simulink model "S4_LP_SCR_bypass_2018b"  (R2018b)
settings: Solver=VariableStepAuto  StartTime=0.0  StopTime=20000  RelTol=1e-3
undefined symbols (not defined in the file or in its folder): sigbuilder_block
libraries: fl_lib x70, sh_lib x49, nesl_utility x29
(part 1 of 2)
settings Model: Creator=USER  LastModifiedBy=USER
settings DataIOCC: ReturnWorkspaceOutputs=on
settings DebuggingCC: UnconnectedInputMsg=none  UnconnectedOutputMsg=none  UnconnectedLineMsg=none  SFMachineParentedDataDiag=error
settings SimscapeCC: SimscapeLogType=all

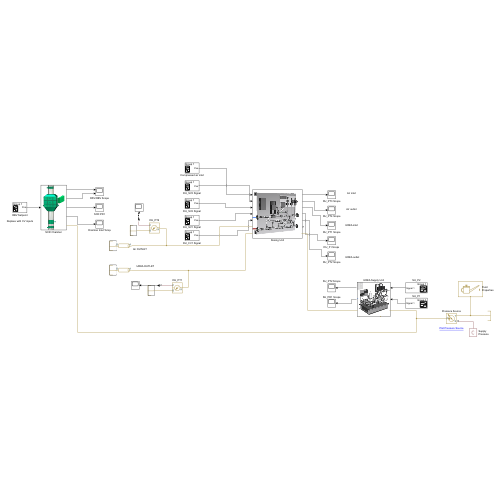
[thumbnail: Simulink's stored preview of the top-level diagram]
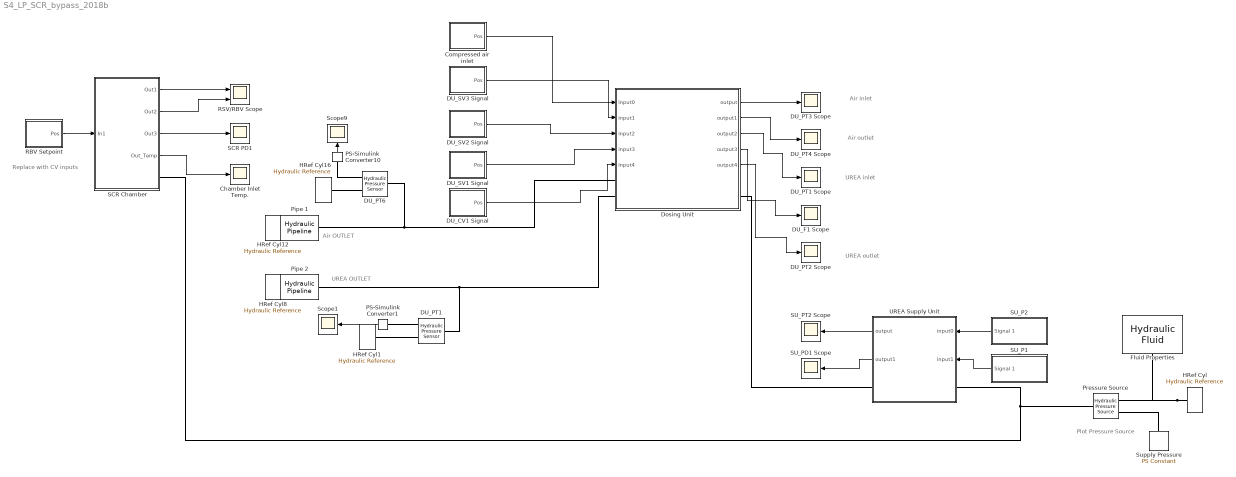
== system S4_LP_SCR_bypass_2018b ==
  note: Air inlet
  note: UREA inlet
  note: UREA outlet
  note: Air outlet
  note: Air OUTLET
  note: Plot Pressure Source
  note: UREA OUTLET
  note: Replace with CV inputs
  Chamber Inlet Temp. : Scope
  Compressed air inlet : Subsystem  Tag=STV Subsys  LoadFcn=sigbuilder_block('load');  StartFcn=sigbuilder_block('start');  StopFcn=sigbuilder_block('stop');  ClipboardFcn=sigbuilder_block('clipboard');  mask(Sigbuilder block){tuvar=[0:10]}
      mask help: Sigbuilder GUI
      mask init:
      | if ~strcmp(get_param(bdroot(gcbh),'SimulationStatus'),'stopped') tuvar = sigbuilder_block('maskInit'); end
      settings: CopyFcn=sigbuilder_block('copy');  DeleteFcn=sigbuilder_block('delete');  ModelCloseFcn=sigbuilder_block('modelClose');  PreSaveFcn=sigbuilder_block('preSave');  PauseFcn=sigbuilder_block('pause')  ContinueFcn=sigbuilder_block('continue')  NameChangeFcn=sigbuilder_block('namechange');  OpenFcn=sigbuilder_block('open',[0 0 787.5 524.25 ]);  CloseFcn=sigbuilder_block('close');
      mask Display: plot(0, 0, 100, 100,[2, 2, 32, 32, 2], [68, 8, 8, 68, 68],[32, 2], [38, 38], [32, 19, 2],[53, 60, 44], [32, 17, 17, 2],[16, 16, 31, 31]);txt = getActiveGroup(gcbh);text(2, 100, txt,'verticalAlignment', 'top');
  DU_CV1 Signal : Subsystem  Tag=STV Subsys  LoadFcn=sigbuilder_block('load');  StartFcn=sigbuilder_block('start');  StopFcn=sigbuilder_block('stop');  ClipboardFcn=sigbuilder_block('clipboard');  mask(Sigbuilder block){tuvar=[0:10]}
      mask help: Sigbuilder GUI
      mask init:
      | if ~strcmp(get_param(bdroot(gcbh),'SimulationStatus'),'stopped') tuvar = sigbuilder_block('maskInit'); end
      settings: CopyFcn=sigbuilder_block('copy');  DeleteFcn=sigbuilder_block('delete');  ModelCloseFcn=sigbuilder_block('modelClose');  PreSaveFcn=sigbuilder_block('preSave');  PauseFcn=sigbuilder_block('pause')  ContinueFcn=sigbuilder_block('continue')  NameChangeFcn=sigbuilder_block('namechange');  OpenFcn=sigbuilder_block('open',[0 0 787.5 524.25 ]);  CloseFcn=sigbuilder_block('close');
      mask Display: plot(0, 0, 100, 100,[2, 2, 32, 32, 2], [68, 8, 8, 68, 68],[32, 2], [38, 38], [32, 19, 2],[53, 60, 44], [32, 17, 17, 2],[16, 16, 31, 31]);txt = getActiveGroup(gcbh);text(2, 100, txt,'verticalAlignment', 'top');
  DU_F1 Scope : Scope
  DU_PT1 : fl_lib/Hydraulic/Hydraulic Sensors/Hydraulic Pressure Sensor
      settings: SourceProductBaseCode=PW,SS,VE
  DU_PT1 Scope : Scope
  DU_PT2 Scope : Scope
  DU_PT3 Scope : Scope
  DU_PT4 Scope : Scope
  DU_PT6 : fl_lib/Hydraulic/Hydraulic Sensors/Hydraulic Pressure Sensor
      settings: SourceProductBaseCode=PW,SS,VE
  DU_SV1 Signal : Subsystem  Tag=STV Subsys  LoadFcn=sigbuilder_block('load');  StartFcn=sigbuilder_block('start');  StopFcn=sigbuilder_block('stop');  ClipboardFcn=sigbuilder_block('clipboard');  mask(Sigbuilder block){tuvar=[0:10]}
      mask help: Sigbuilder GUI
      mask init:
      | if ~strcmp(get_param(bdroot(gcbh),'SimulationStatus'),'stopped') tuvar = sigbuilder_block('maskInit'); end
      settings: CopyFcn=sigbuilder_block('copy');  DeleteFcn=sigbuilder_block('delete');  ModelCloseFcn=sigbuilder_block('modelClose');  PreSaveFcn=sigbuilder_block('preSave');  PauseFcn=sigbuilder_block('pause')  ContinueFcn=sigbuilder_block('continue')  NameChangeFcn=sigbuilder_block('namechange');  OpenFcn=sigbuilder_block('open',[0 0 787.5 524.25 ]);  CloseFcn=sigbuilder_block('close');
      mask Display: plot(0, 0, 100, 100,[2, 2, 32, 32, 2], [68, 8, 8, 68, 68],[32, 2], [38, 38], [32, 19, 2],[53, 60, 44], [32, 17, 17, 2],[16, 16, 31, 31]);txt = getActiveGroup(gcbh);text(2, 100, txt,'verticalAlignment', 'top');
  DU_SV2 Signal : Subsystem  Tag=STV Subsys  LoadFcn=sigbuilder_block('load');  StartFcn=sigbuilder_block('start');  StopFcn=sigbuilder_block('stop');  ClipboardFcn=sigbuilder_block('clipboard');  mask(Sigbuilder block){tuvar=[0:10]}
      mask help: Sigbuilder GUI
      mask init:
      | if ~strcmp(get_param(bdroot(gcbh),'SimulationStatus'),'stopped') tuvar = sigbuilder_block('maskInit'); end
      settings: CopyFcn=sigbuilder_block('copy');  DeleteFcn=sigbuilder_block('delete');  ModelCloseFcn=sigbuilder_block('modelClose');  PreSaveFcn=sigbuilder_block('preSave');  PauseFcn=sigbuilder_block('pause')  ContinueFcn=sigbuilder_block('continue')  NameChangeFcn=sigbuilder_block('namechange');  OpenFcn=sigbuilder_block('open',[0 0 787.5 524.25 ]);  CloseFcn=sigbuilder_block('close');
      mask Display: plot(0, 0, 100, 100,[2, 2, 32, 32, 2], [68, 8, 8, 68, 68],[32, 2], [38, 38], [32, 19, 2],[53, 60, 44], [32, 17, 17, 2],[16, 16, 31, 31]);txt = getActiveGroup(gcbh);text(2, 100, txt,'verticalAlignment', 'top');
  DU_SV3 Signal : Subsystem  Tag=STV Subsys  LoadFcn=sigbuilder_block('load');  StartFcn=sigbuilder_block('start');  StopFcn=sigbuilder_block('stop');  ClipboardFcn=sigbuilder_block('clipboard');  mask(Sigbuilder block){tuvar=[0:10]}
      mask help: Sigbuilder GUI
      mask init:
      | if ~strcmp(get_param(bdroot(gcbh),'SimulationStatus'),'stopped') tuvar = sigbuilder_block('maskInit'); end
      settings: CopyFcn=sigbuilder_block('copy');  DeleteFcn=sigbuilder_block('delete');  ModelCloseFcn=sigbuilder_block('modelClose');  PreSaveFcn=sigbuilder_block('preSave');  PauseFcn=sigbuilder_block('pause')  ContinueFcn=sigbuilder_block('continue')  NameChangeFcn=sigbuilder_block('namechange');  OpenFcn=sigbuilder_block('open',[1483.5 44.25 813 562.5 ]);  CloseFcn=sigbuilder_block('close');
      mask Display: plot(0, 0, 100, 100,[2, 2, 32, 32, 2], [68, 8, 8, 68, 68],[32, 2], [38, 38], [32, 19, 2],[53, 60, 44], [32, 17, 17, 2],[16, 16, 31, 31]);txt = getActiveGroup(gcbh);text(2, 100, txt,'verticalAlignment', 'top');
  Dosing Unit : Subsystem
      mask Display: image('DosingUnit.png')
  Fluid Properties : sh_lib/Hydraulic Utilities/Hydraulic Fluid  Tag=Factory Generic  SelFluid=2  SysTemp=40  TrapAir=0.001  ViscDerFactor=1  range_error=2
  HRef Cyl{,1,8,12,16} (5 alike) : fl_lib/Hydraulic/Hydraulic Elements/Hydraulic Reference  Tag=Factory Generic
      settings: SourceProductBaseCode=PW,SS,VE
  PS-Simulink Converter1 : nesl_utility/PS-Simulink Converter  PhysicalDomain=network_engine_domain  SubClassName=ps_output  LeftPortType=input  RightPortType=output  PseudoPeriodic=off  Frequencies=[]  VectorFormat=inherit  Unit=inherit  AffineConversion=off
      settings: SourceProductBaseCode=SS,PW,VE
  PS-Simulink Converter10 : nesl_utility/PS-Simulink Converter  PhysicalDomain=network_engine_domain  SubClassName=ps_output  LeftPortType=input  RightPortType=output  PseudoPeriodic=off  Frequencies=[]  VectorFormat=inherit  Unit=inherit  AffineConversion=off
      settings: SourceProductBaseCode=SS,PW,VE
  Pipe 1 : sh_lib/Pipelines/Hydraulic Pipeline  Tag=Factory Generic  cs_type=1  d_in=0.1 m  area=1e-04 m^2  D_h=0.0112 m  s_factor=64  length=5 m  length_ad=1 m  roughness=1.5e-05 m  Re_lam=2e+03  Re_turb=4e+03  wall_type=1  pr_r_coef=2e-10 m/Pa  time_const=0.008 s  k_sh=1.4  initial_pressure=0 Pa
      settings: SourceProductBaseCode=SH  InternalSimscapePortConfiguration="{\"Bottom\":[],\"Left\":[{\"id\":\"A\",\"label\":\"A\",\"type\":\"foundation.hydraulic.hydraulic\"}],\"Right\":[{\"id\":\"B\",\"label\":\"B\",\"type\":\"foundation.hydraulic.hydraulic\"}],\"Top\":[]}"
  Pipe 2 : sh_lib/Pipelines/Hydraulic Pipeline  Tag=Factory Generic  cs_type=1  d_in=0.1 m  area=1e-04 m^2  D_h=0.0112 m  s_factor=64  length=1 m  length_ad=1 m  roughness=1.5e-05 m  Re_lam=2e+03  Re_turb=4e+03  wall_type=1  pr_r_coef=2e-10 m/Pa  time_const=0.008 s  k_sh=1.4  initial_pressure=0 Pa
      settings: SourceProductBaseCode=SH  InternalSimscapePortConfiguration="{\"Bottom\":[],\"Left\":[{\"id\":\"A\",\"label\":\"A\",\"type\":\"foundation.hydraulic.hydraulic\"}],\"Right\":[{\"id\":\"B\",\"label\":\"B\",\"type\":\"foundation.hydraulic.hydraulic\"}],\"Top\":[]}"
  Pressure Source : fl_lib/Hydraulic/Hydraulic Sources/Hydraulic Pressure Source  Tag=Factory Generic
      settings: SourceProductBaseCode=PW,SS,VE  InternalSimscapePortConfiguration="{\"Bottom\":[],\"Left\":[{\"id\":\"P\",\"label\":\"P\",\"type\":\"foundation.hydraulic.hydraulic\"}],\"Right\":[{\"id\":\"S\",\"label\":\"S\",\"type\":\"input\"},{\"id\":\"T\",\"label\":\"T\",\"type\":\"foundation.hydraulic.hydraulic\"}],\"Top\":[]}"
  RBV Setpoint : Subsystem  Tag=STV Subsys  LoadFcn=sigbuilder_block('load');  StartFcn=sigbuilder_block('start');  StopFcn=sigbuilder_block('stop');  ClipboardFcn=sigbuilder_block('clipboard');  mask(Sigbuilder block){tuvar=[0:10]}
      mask help: Sigbuilder GUI
      mask init:
      | if ~strcmp(get_param(bdroot(gcbh),'SimulationStatus'),'stopped') tuvar = sigbuilder_block('maskInit'); end
      settings: CopyFcn=sigbuilder_block('copy');  DeleteFcn=sigbuilder_block('delete');  ModelCloseFcn=sigbuilder_block('modelClose');  PreSaveFcn=sigbuilder_block('preSave');  PauseFcn=sigbuilder_block('pause')  ContinueFcn=sigbuilder_block('continue')  NameChangeFcn=sigbuilder_block('namechange');  OpenFcn=sigbuilder_block('open',[0 0 787.5 524.25 ]);  CloseFcn=sigbuilder_block('close');
      mask Display: plot(0, 0, 100, 100,[2, 2, 32, 32, 2], [68, 8, 8, 68, 68],[32, 2], [38, 38], [32, 19, 2],[53, 60, 44], [32, 17, 17, 2],[16, 16, 31, 31]);txt = getActiveGroup(gcbh);text(2, 100, txt,'verticalAlignment', 'top');
  RSV/RBV Scope : Scope  NumInputPorts=2
  SCR Chamber : Subsystem
      mask Display: image('SCRChamber.png')
  SCR PD1 : Scope
  SU_P1 : Subsystem  Tag=STV Subsys  LoadFcn=sigbuilder_block('load');  StartFcn=sigbuilder_block('start');  StopFcn=sigbuilder_block('stop');  ClipboardFcn=sigbuilder_block('clipboard');  mask(Sigbuilder block){tuvar=[0:10]}
      mask help: Simulink:masks:SigbuilderBlock_MD
      mask init:
      | if ~strcmp(get_param(bdroot(gcbh),'SimulationStatus'),'stopped') tuvar = sigbuilder_block('maskInit'); end
      settings: CopyFcn=sigbuilder_block('copy');  DeleteFcn=sigbuilder_block('delete');  ModelCloseFcn=sigbuilder_block('modelClose');  PreSaveFcn=sigbuilder_block('preSave');  PauseFcn=sigbuilder_block('pause');  ContinueFcn=sigbuilder_block('continue');  NameChangeFcn=sigbuilder_block('namechange');  OpenFcn=sigbuilder_block('open',[0 0 787.5 524.25 ]);  CloseFcn=sigbuilder_block('close');
      mask Display: plot(0, 0, 100, 100,[2, 2, 32, 32, 2], [68, 8, 8, 68, 68],[32, 2], [38, 38], [32, 19, 2],[53, 60, 44], [32, 17, 17, 2],[16, 16, 31, 31]);txt = getActiveGroup(gcbh);text(2, 100, txt,'verticalAlignment', 'top');
  SU_P2 : Subsystem  Tag=STV Subsys  LoadFcn=sigbuilder_block('load');  StartFcn=sigbuilder_block('start');  StopFcn=sigbuilder_block('stop');  ClipboardFcn=sigbuilder_block('clipboard');  mask(Sigbuilder block){tuvar=[0:10]}
      mask help: Simulink:masks:SigbuilderBlock_MD
      mask init:
      | if ~strcmp(get_param(bdroot(gcbh),'SimulationStatus'),'stopped') tuvar = sigbuilder_block('maskInit'); end
      settings: CopyFcn=sigbuilder_block('copy');  DeleteFcn=sigbuilder_block('delete');  ModelCloseFcn=sigbuilder_block('modelClose');  PreSaveFcn=sigbuilder_block('preSave');  PauseFcn=sigbuilder_block('pause');  ContinueFcn=sigbuilder_block('continue');  NameChangeFcn=sigbuilder_block('namechange');  OpenFcn=sigbuilder_block('open',[0 0 787.5 524.25 ]);  CloseFcn=sigbuilder_block('close');
      mask Display: plot(0, 0, 100, 100,[2, 2, 32, 32, 2], [68, 8, 8, 68, 68],[32, 2], [38, 38], [32, 19, 2],[53, 60, 44], [32, 17, 17, 2],[16, 16, 31, 31]);txt = getActiveGroup(gcbh);text(2, 100, txt,'verticalAlignment', 'top');
  SU_PD1 Scope : Scope
  SU_PT2 Scope : Scope
  Scope1 : Scope
  Scope9 : Scope
  Supply Pressure : fl_lib/Physical Signals/Sources/PS Constant  constant=7 Pa
      settings: SourceProductBaseCode=PW,SS,VE
  UREA Supply Unit : Subsystem
      mask Display: image('UreaSupplyUnit.png')
  wires:
  SU_P2/1(Signal 1) -> UREA Supply Unit/1(input0)
  SU_P1/1(Signal 1) -> UREA Supply Unit/2(input1)
  UREA Supply Unit/1(output) -> SU_PT2 Scope/1
  UREA Supply Unit/2(output1) -> SU_PD1 Scope/1
  Compressed air inlet/1(Pos) -> Dosing Unit/1(input0)
  DU_SV3 Signal/1(Pos) -> Dosing Unit/2(input1)
  DU_SV2 Signal/1(Pos) -> Dosing Unit/3(input2)
  DU_SV1 Signal/1(Pos) -> Dosing Unit/4(input3)
  DU_CV1 Signal/1(Pos) -> Dosing Unit/5(input4)
  Dosing Unit/1(output) -> DU_PT3 Scope/1
  Dosing Unit/2(output1) -> DU_PT4 Scope/1
  Dosing Unit/3(output2) -> DU_PT1 Scope/1
  Dosing Unit/4(output3) -> DU_F1 Scope/1
  Dosing Unit/5(output4) -> DU_PT2 Scope/1
  PS-Simulink Converter10/1 -> Scope9/1
  PS-Simulink Converter1/1 -> Scope1/1
  RBV Setpoint/1(Pos) -> SCR Chamber/1(In1)
  SCR Chamber/1(Out1) -> RSV/RBV Scope/1
  SCR Chamber/2(Out2) -> RSV/RBV Scope/2
  SCR Chamber/3(Out3) -> SCR PD1/1
  SCR Chamber/4(Out_Temp) -> Chamber Inlet Temp./1
  connections:
  HRef Cyl/LConn1 -- Fluid Properties/RConn1 -- Pressure Source/RConn2
  Supply Pressure/RConn1 -- Pressure Source/RConn1
  Pipe 1/RConn1 -- HRef Cyl12/LConn1
  Pipe 2/RConn1 -- HRef Cyl8/LConn1
  Pipe 1/LConn1 -- DU_PT6/LConn1 -- Dosing Unit/LConn1
  Dosing Unit/LConn2 -- Pipe 2/LConn1 -- DU_PT1/LConn1
  UREA Supply Unit/RConn1 -- Dosing Unit/RConn2
  PS-Simulink Converter10/LConn1 -- DU_PT6/RConn2
  HRef Cyl16/LConn1 -- DU_PT6/RConn1
  HRef Cyl1/LConn1 -- DU_PT1/RConn1
  PS-Simulink Converter1/LConn1 -- DU_PT1/RConn2
  Pressure Source/LConn1 -- SCR Chamber/RConn1 -- UREA Supply Unit/LConn1

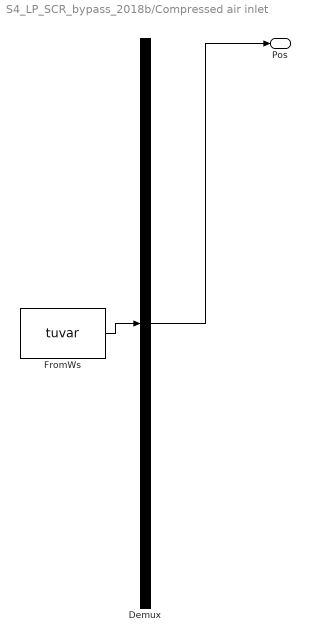
== system S4_LP_SCR_bypass_2018b/Compressed air inlet ==
  Demux : Demux  Tag=STV Demux  Outputs=1
      settings: DisplayOption=none
  FromWs : FromWorkspace  Tag=STV FromWs  VariableName=tuvar
      SigBuilderData=|
      | common.afterFinalStr = 'Extrapolate'
      | common.sampleTime = 0
      | dataSet.timeRange = [0 20000]
      | dataSet.name = 'Group 1'
      | sbobj.Groups.Name = 'Group 1'
      | sbobj.Groups.Signals.Name = 'Pos'
      | sbobj.Groups.Signals.XData = [0 20000]
      | sbobj.Groups.Signals.YData = [1 1]
      | sbobj.Groups.TimeRange = [0 20000]
  Pos : Outport  Tag=STV Outport  VectorParamsAs1DForOutWhenUnconnected=off
  wires:
  Demux/1 -> Pos/1
  FromWs/1 -> Demux/1

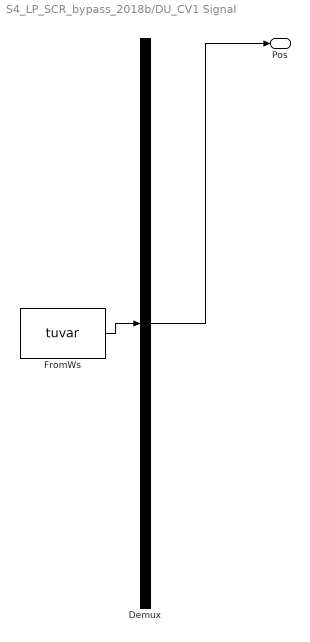
== system S4_LP_SCR_bypass_2018b/DU_CV1 Signal ==
  Demux : Demux  Tag=STV Demux  Outputs=1
      settings: DisplayOption=none
  FromWs : FromWorkspace  Tag=STV FromWs  VariableName=tuvar
      SigBuilderData=|
      | common.afterFinalStr = 'Extrapolate'
      | common.sampleTime = 0
      | dataSet.timeRange = [0 20000]
      | dataSet.name = 'Group 1'
      | sbobj.Groups.Name = 'Group 1'
      | sbobj.Groups.Signals.Name = 'Pos'
      | sbobj.Groups.Signals.XData = [0 8720 8720 9040 9040 11820 11820 12436 12436 20000]
      | sbobj.Groups.Signals.YData = [0 0 1 1 -0.005 0 1 1 0 0]
      | sbobj.Groups.TimeRange = [0 20000]
  Pos : Outport  Tag=STV Outport  VectorParamsAs1DForOutWhenUnconnected=off
  wires:
  Demux/1 -> Pos/1
  FromWs/1 -> Demux/1

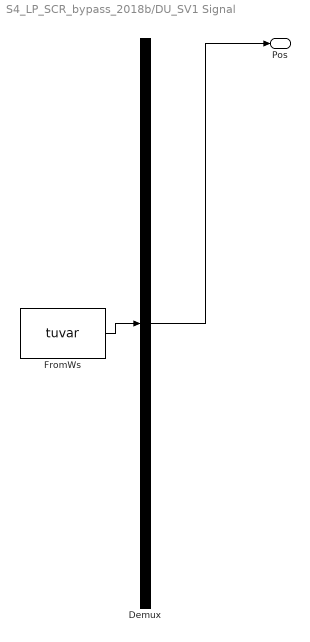
== system S4_LP_SCR_bypass_2018b/DU_SV1 Signal ==
  Demux : Demux  Tag=STV Demux  Outputs=1
      settings: DisplayOption=none
  FromWs : FromWorkspace  Tag=STV FromWs  VariableName=tuvar
      SigBuilderData=|
      | common.afterFinalStr = 'Extrapolate'
      | common.sampleTime = 0
      | dataSet.timeRange = [0 20000]
      | dataSet.name = 'Group 1'
      | sbobj.Groups.Name = 'Group 1'
      | sbobj.Groups.Signals.Name = 'Pos'
      | sbobj.Groups.Signals.XData = [0 9040 9040 11820 11820 20000]
      | sbobj.Groups.Signals.YData = [0 0 1 1 0 0]
      | sbobj.Groups.TimeRange = [0 20000]
  Pos : Outport  Tag=STV Outport  VectorParamsAs1DForOutWhenUnconnected=off
  wires:
  Demux/1 -> Pos/1
  FromWs/1 -> Demux/1

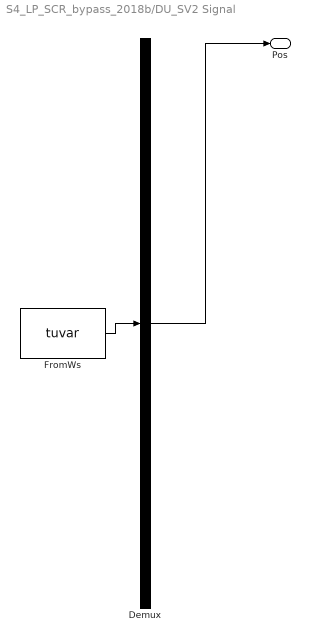
== system S4_LP_SCR_bypass_2018b/DU_SV2 Signal ==
  Demux : Demux  Tag=STV Demux  Outputs=1
      settings: DisplayOption=none
  FromWs : FromWorkspace  Tag=STV FromWs  VariableName=tuvar
      SigBuilderData=|
      | common.afterFinalStr = 'Extrapolate'
      | common.sampleTime = 0
      | dataSet.timeRange = [0 20000]
      | dataSet.name = 'Group 1'
      | sbobj.Groups.Name = 'Group 1'
      | sbobj.Groups.Signals.Name = 'Pos'
      | sbobj.Groups.Signals.XData = [0 8720 8720 9040 9040 11820 11820 12436 12436 20000]
      | sbobj.Groups.Signals.YData = [0 0 1 1 -0.005 0 1 1 0 0]
      | sbobj.Groups.TimeRange = [0 20000]
  Pos : Outport  Tag=STV Outport  VectorParamsAs1DForOutWhenUnconnected=off
  wires:
  Demux/1 -> Pos/1
  FromWs/1 -> Demux/1

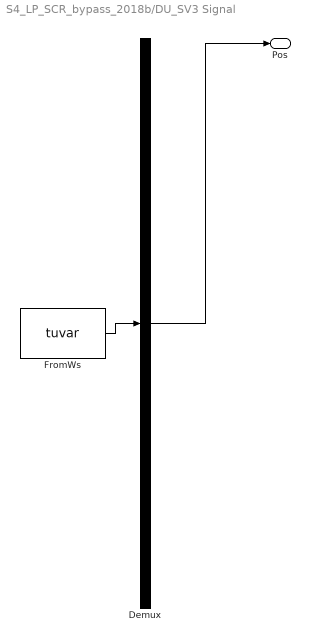
== system S4_LP_SCR_bypass_2018b/DU_SV3 Signal ==
  Demux : Demux  Tag=STV Demux  Outputs=1
      settings: DisplayOption=none
  FromWs : FromWorkspace  Tag=STV FromWs  VariableName=tuvar
      SigBuilderData=|
      | common.afterFinalStr = 'Extrapolate'
      | common.sampleTime = 0
      | dataSet.timeRange = [0 20000]
      | dataSet.name = 'Group 1'
      | sbobj.Groups.Name = 'Group 1'
      | sbobj.Groups.Signals.Name = 'Pos'
      | sbobj.Groups.Signals.XData = [0 8696 8696 12251 12251 20000]
      | sbobj.Groups.Signals.YData = [0 0 1 1 0 0]
      | sbobj.Groups.TimeRange = [0 20000]
  Pos : Outport  Tag=STV Outport  VectorParamsAs1DForOutWhenUnconnected=off
  wires:
  Demux/1 -> Pos/1
  FromWs/1 -> Demux/1

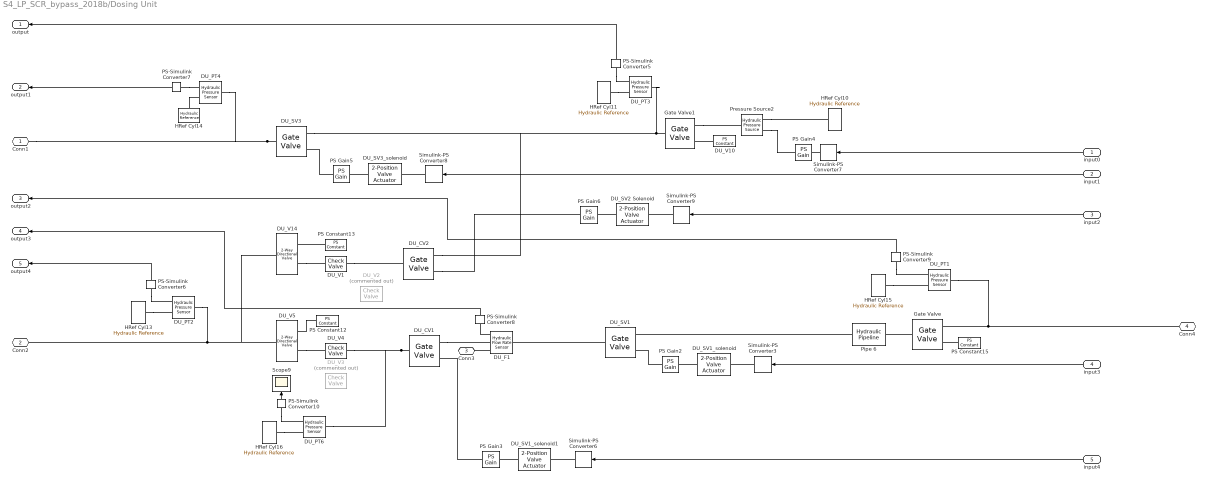
== system S4_LP_SCR_bypass_2018b/Dosing Unit ==
  input0 : Inport
  input1 : Inport  Port=2
  input2 : Inport  Port=3
  input3 : Inport  Port=4
  input4 : Inport  Port=5
  DU_CV1 : sh_lib/Valves/Flow Control Valves/Gate Valve  d_gate=0.1 m  x_0=0 m  C_d=1e3  A_leak=500 m^2  lam_spec=1  B_lam=0.999  Re_cr=10
      settings: SourceProductBaseCode=SH  InternalSimscapePortConfiguration="{\"Bottom\":[],\"Left\":[{\"id\":\"S\",\"label\":\"S\",\"type\":\"input\"},{\"id\":\"A\",\"label\":\"A\",\"type\":\"foundation.hydraulic.hydraulic\"}],\"Right\":[{\"id\":\"B\",\"label\":\"B\",\"type\":\"foundation.hydraulic.hydraulic\"}],\"Top\":[]}"
  DU_CV2 : sh_lib/Valves/Flow Control Valves/Gate Valve  d_gate=0.1 m  x_0=0 m  C_d=1e3  A_leak=500 m^2  lam_spec=1  B_lam=0.999  Re_cr=10
      settings: SourceProductBaseCode=SH  InternalSimscapePortConfiguration="{\"Bottom\":[],\"Left\":[{\"id\":\"S\",\"label\":\"S\",\"type\":\"input\"},{\"id\":\"A\",\"label\":\"A\",\"type\":\"foundation.hydraulic.hydraulic\"}],\"Right\":[{\"id\":\"B\",\"label\":\"B\",\"type\":\"foundation.hydraulic.hydraulic\"}],\"Top\":[]}"
  DU_F1 : fl_lib/Hydraulic/Hydraulic Sensors/Hydraulic Flow Rate Sensor
      settings: SourceProductBaseCode=PW,SS,VE
  DU_PT{1..4,6} (5 alike) : fl_lib/Hydraulic/Hydraulic Sensors/Hydraulic Pressure Sensor
      settings: SourceProductBaseCode=PW,SS,VE
  DU_SV1 : sh_lib/Valves/Flow Control Valves/Gate Valve  d_gate=0.1 m  x_0=0 m  C_d=500  A_leak=1e-20 m^2  lam_spec=1  B_lam=0.999  Re_cr=10
      settings: SourceProductBaseCode=SH  InternalSimscapePortConfiguration="{\"Bottom\":[],\"Left\":[{\"id\":\"S\",\"label\":\"S\",\"type\":\"input\"},{\"id\":\"A\",\"label\":\"A\",\"type\":\"foundation.hydraulic.hydraulic\"}],\"Right\":[{\"id\":\"B\",\"label\":\"B\",\"type\":\"foundation.hydraulic.hydraulic\"}],\"Top\":[]}"
  DU_SV1_solenoid : sh_lib/Valves/Valve Actuators/2-Position Valve Actuator  stroke=1 m  t_on=2 s  t_off=2 s  act_signal=1e-20  init_position=0  act_orientation=1
      settings: SourceProductBaseCode=SH  InternalSimscapePortConfiguration="{\"Bottom\":[],\"Left\":[{\"id\":\"C\",\"label\":\"\",\"type\":\"input\"}],\"Right\":[{\"id\":\"P\",\"label\":\"\",\"type\":\"output\"}],\"Top\":[]}"
  DU_SV1_solenoid1 : sh_lib/Valves/Valve Actuators/2-Position Valve Actuator  stroke=1 m  t_on=2 s  t_off=2 s  act_signal=1e-20  init_position=0  act_orientation=1
      settings: SourceProductBaseCode=SH  InternalSimscapePortConfiguration="{\"Bottom\":[],\"Left\":[{\"id\":\"C\",\"label\":\"\",\"type\":\"input\"}],\"Right\":[{\"id\":\"P\",\"label\":\"\",\"type\":\"output\"}],\"Top\":[]}"
  DU_SV2 Solenoid : sh_lib/Valves/Valve Actuators/2-Position Valve Actuator  stroke=1 m  t_on=2 s  t_off=2 s  act_signal=1e-20  init_position=0  act_orientation=1
      settings: SourceProductBaseCode=SH  InternalSimscapePortConfiguration="{\"Bottom\":[],\"Left\":[{\"id\":\"C\",\"label\":\"\",\"type\":\"input\"}],\"Right\":[{\"id\":\"P\",\"label\":\"\",\"type\":\"output\"}],\"Top\":[]}"
  DU_SV3 : sh_lib/Valves/Flow Control Valves/Gate Valve  d_gate=0.1 m  x_0=0 m  C_d=500  A_leak=1e-20 m^2  lam_spec=1  B_lam=0.999  Re_cr=10
      settings: SourceProductBaseCode=SH  InternalSimscapePortConfiguration="{\"Bottom\":[],\"Left\":[{\"id\":\"S\",\"label\":\"S\",\"type\":\"input\"},{\"id\":\"A\",\"label\":\"A\",\"type\":\"foundation.hydraulic.hydraulic\"}],\"Right\":[{\"id\":\"B\",\"label\":\"B\",\"type\":\"foundation.hydraulic.hydraulic\"}],\"Top\":[]}"
  DU_SV3_solenoid : sh_lib/Valves/Valve Actuators/2-Position Valve Actuator  stroke=1 m  t_on=2 s  t_off=2 s  act_signal=1e-20  init_position=0  act_orientation=1
      settings: SourceProductBaseCode=SH  InternalSimscapePortConfiguration="{\"Bottom\":[],\"Left\":[{\"id\":\"C\",\"label\":\"\",\"type\":\"input\"}],\"Right\":[{\"id\":\"P\",\"label\":\"\",\"type\":\"output\"}],\"Top\":[]}"
  DU_V1 : sh_lib/Valves/Directional Valves/Check Valve  area_max=1e-4 m^2  pres_crack=1e-4 Pa  pres_max=1.2e5 Pa  C_d=0.7  A_leak=1e-12 m^2  lam_spec=1  B_lam=0.999  Re_cr=12  dynamic=0  tau=0.1 s  area_init=1e-12 m^2
      settings: SourceProductBaseCode=SH  InternalSimscapePortConfiguration="{\"Bottom\":[],\"Left\":[{\"id\":\"A\",\"label\":\"A\",\"type\":\"foundation.hydraulic.hydraulic\"}],\"Right\":[{\"id\":\"B\",\"label\":\"B\",\"type\":\"foundation.hydraulic.hydraulic\"}],\"Top\":[]}"
  DU_V10 : fl_lib/Physical Signals/Sources/PS Constant  constant=0.1
      settings: SourceProductBaseCode=PW,SS,VE
  DU_V14 : sh_lib/Valves/Directional Valves/2-Way Directional Valve  Tag=Factory Generic  mdl_type=1  area_max=0.1 m^2  opening_max=0.01 m  opening_tab="[  -0.002 0 0.005 0.015 ] m"  area_tab="[  1e-12 4e-12 1e-05 1.02e-05 ] m^2"  pressure_tab="[  -5e+06 -2e+06 2e+06 5e+06 ] Pa"  flow_rate_tab="[  -1e-12 -6e-14 6e+12 1e+11 ; -8e-08 -4e-08 4e+06 8e+06 ; -0.0025 -0.00103 0.001 0.0024 ; -0.00258 -0.001032 0.00106 0.00247 ; ] m^3/s"  interp_method=1  extrap_method=1  C_d=500  x_0=8.0e-4 m  A_leak=1e-12 m^2  lam_spec=1  B_lam=0.999  Re_cr=12
      settings: SourceProductBaseCode=SH  LogSimulationData=on  InternalSimscapePortConfiguration="{\"Bottom\":[],\"Left\":[{\"id\":\"S\",\"label\":\"S\",\"type\":\"input\"},{\"id\":\"A\",\"label\":\"A\",\"type\":\"foundation.hydraulic.hydraulic\"}],\"Right\":[{\"id\":\"B\",\"label\":\"B\",\"type\":\"foundation.hydraulic.hydraulic\"}],\"Top\":[]}"
  DU_V2 : sh_lib/Valves/Directional Valves/Check Valve  Commented=on  area_max=1e-4 m^2  pres_crack=0.3e5 Pa  pres_max=1.2e5 Pa  C_d=500  A_leak=1e-12 m^2  lam_spec=1  B_lam=0.999  Re_cr=12  dynamic=0  tau=0.1 s  area_init=1e-12 m^2
      settings: SourceProductBaseCode=SH  InternalSimscapePortConfiguration="{\"Bottom\":[],\"Left\":[{\"id\":\"A\",\"label\":\"A\",\"type\":\"foundation.hydraulic.hydraulic\"}],\"Right\":[{\"id\":\"B\",\"label\":\"B\",\"type\":\"foundation.hydraulic.hydraulic\"}],\"Top\":[]}"
  DU_V3 : sh_lib/Valves/Directional Valves/Check Valve  Commented=on  area_max=0.01 m^2  pres_crack=3e+04 Pa  pres_max=1.2e5 Pa  C_d=500  A_leak=1e-12 m^2  lam_spec=1  B_lam=0.999  Re_cr=12  dynamic=0  tau=0.1 s  area_init=1e-12 m^2
      settings: SourceProductBaseCode=SH  InternalSimscapePortConfiguration="{\"Bottom\":[],\"Left\":[{\"id\":\"A\",\"label\":\"A\",\"type\":\"foundation.hydraulic.hydraulic\"}],\"Right\":[{\"id\":\"B\",\"label\":\"B\",\"type\":\"foundation.hydraulic.hydraulic\"}],\"Top\":[]}"
  DU_V4 : sh_lib/Valves/Directional Valves/Check Valve  area_max=0.01 m^2  pres_crack=1e-4 Pa  pres_max=1 Pa  C_d=500  A_leak=1e-12 m^2  lam_spec=1  B_lam=0.999  Re_cr=12  dynamic=0  tau=0.1 s  area_init=1e-12 m^2
      settings: SourceProductBaseCode=SH  InternalSimscapePortConfiguration="{\"Bottom\":[],\"Left\":[{\"id\":\"A\",\"label\":\"A\",\"type\":\"foundation.hydraulic.hydraulic\"}],\"Right\":[{\"id\":\"B\",\"label\":\"B\",\"type\":\"foundation.hydraulic.hydraulic\"}],\"Top\":[]}"
  DU_V5 : sh_lib/Valves/Directional Valves/2-Way Directional Valve  Tag=Factory Generic  mdl_type=1  area_max=0.1 m^2  opening_max=0.01 m  opening_tab="[  -0.002 0 0.005 0.015 ] m"  area_tab="[  1e-12 4e-12 1e-05 1.02e-05 ] m^2"  pressure_tab="[  -5e+06 -2e+06 2e+06 5e+06 ] Pa"  flow_rate_tab="[  -1e-12 -6e-14 6e+12 1e+11 ; -8e-08 -4e-08 4e+06 8e+06 ; -0.0025 -0.00103 0.001 0.0024 ; -0.00258 -0.001032 0.00106 0.00247 ; ] m^3/s"  interp_method=1  extrap_method=1  C_d=500  x_0=8.0e-4 m  A_leak=1e-12 m^2  lam_spec=1  B_lam=0.999  Re_cr=12
      settings: SourceProductBaseCode=SH  LogSimulationData=on  InternalSimscapePortConfiguration="{\"Bottom\":[],\"Left\":[{\"id\":\"S\",\"label\":\"S\",\"type\":\"input\"},{\"id\":\"A\",\"label\":\"A\",\"type\":\"foundation.hydraulic.hydraulic\"}],\"Right\":[{\"id\":\"B\",\"label\":\"B\",\"type\":\"foundation.hydraulic.hydraulic\"}],\"Top\":[]}"
  Gate Valve : sh_lib/Valves/Flow Control Valves/Gate Valve  d_gate=0.1 m  x_0=0 m  C_d=500  A_leak=1e-20 m^2  lam_spec=1  B_lam=0.99  Re_cr=10
      settings: SourceProductBaseCode=SH  InternalSimscapePortConfiguration="{\"Bottom\":[],\"Left\":[{\"id\":\"S\",\"label\":\"S\",\"type\":\"input\"},{\"id\":\"A\",\"label\":\"A\",\"type\":\"foundation.hydraulic.hydraulic\"}],\"Right\":[{\"id\":\"B\",\"label\":\"B\",\"type\":\"foundation.hydraulic.hydraulic\"}],\"Top\":[]}"
  Gate Valve1 : sh_lib/Valves/Flow Control Valves/Gate Valve  d_gate=0.1 m  x_0=0 m  C_d=500  A_leak=1e-20 m^2  lam_spec=1  B_lam=0.99  Re_cr=10
      settings: SourceProductBaseCode=SH  InternalSimscapePortConfiguration="{\"Bottom\":[],\"Left\":[{\"id\":\"S\",\"label\":\"S\",\"type\":\"input\"},{\"id\":\"A\",\"label\":\"A\",\"type\":\"foundation.hydraulic.hydraulic\"}],\"Right\":[{\"id\":\"B\",\"label\":\"B\",\"type\":\"foundation.hydraulic.hydraulic\"}],\"Top\":[]}"
  HRef Cyl{10..11,13..16} (6 alike) : fl_lib/Hydraulic/Hydraulic Elements/Hydraulic Reference  Tag=Factory Generic
      settings: SourceProductBaseCode=PW,SS,VE
  PS Constant12 : fl_lib/Physical Signals/Sources/PS Constant  constant=1
      settings: SourceProductBaseCode=PW,SS,VE
  PS Constant13 : fl_lib/Physical Signals/Sources/PS Constant  constant=1
      settings: SourceProductBaseCode=PW,SS,VE
  PS Constant15 : fl_lib/Physical Signals/Sources/PS Constant  constant=0.01
      settings: SourceProductBaseCode=PW,SS,VE
  PS Gain{2..3,5..6} (4 alike) : fl_lib/Physical Signals/Functions/PS Gain  gain=0.1
      settings: SourceProductBaseCode=PW,SS,VE
  PS Gain4 : fl_lib/Physical Signals/Functions/PS Gain  gain=7
      settings: SourceProductBaseCode=PW,SS,VE
  PS-Simulink Converter{5..10} (6 alike) : nesl_utility/PS-Simulink Converter  PhysicalDomain=network_engine_domain  SubClassName=ps_output  LeftPortType=input  RightPortType=output  PseudoPeriodic=off  Frequencies=[]  VectorFormat=inherit  Unit=inherit  AffineConversion=off
      settings: SourceProductBaseCode=SS,PW,VE
  Pipe 6 : sh_lib/Pipelines/Hydraulic Pipeline  Tag=Factory Generic  cs_type=1  d_in=0.016 m  area=1e-04 m^2  D_h=0.0112 m  s_factor=500  length=5 m  length_ad=1 m  roughness=1.5e-05 m  Re_lam=2e+03  Re_turb=4e+03  wall_type=1  pr_r_coef=2e-10 m/Pa  time_const=0.008 s  k_sh=1.4  initial_pressure=0 Pa
      settings: SourceProductBaseCode=SH  LogSimulationData=on  InternalSimscapePortConfiguration="{\"Bottom\":[],\"Left\":[{\"id\":\"A\",\"label\":\"A\",\"type\":\"foundation.hydraulic.hydraulic\"}],\"Right\":[{\"id\":\"B\",\"label\":\"B\",\"type\":\"foundation.hydraulic.hydraulic\"}],\"Top\":[]}"
  Pressure Source2 : fl_lib/Hydraulic/Hydraulic Sources/Hydraulic Pressure Source  Tag=Factory Generic
      settings: SourceProductBaseCode=PW,SS,VE  InternalSimscapePortConfiguration="{\"Bottom\":[],\"Left\":[{\"id\":\"P\",\"label\":\"P\",\"type\":\"foundation.hydraulic.hydraulic\"}],\"Right\":[{\"id\":\"S\",\"label\":\"S\",\"type\":\"input\"},{\"id\":\"T\",\"label\":\"T\",\"type\":\"foundation.hydraulic.hydraulic\"}],\"Top\":[]}"
  Scope9 : Scope
  Simulink-PS Converter{3,6,8..9} (4 alike) : nesl_utility/Simulink-PS Converter  PhysicalDomain=network_engine_domain  SubClassName=ps_input  LeftPortType=input  RightPortType=output  PseudoPeriodic=off  Frequencies=[]  NoiseDistribution=none  NoiseParameters=[]  Unit=m  AffineConversion=off  FilteringAndDerivatives=zero  SimscapeFilterOrder=1  InputFilterTimeConstant=.001  UdotUserProvided=0
      settings: SourceProductBaseCode=SS,PW,VE
  Simulink-PS Converter7 : nesl_utility/Simulink-PS Converter  PhysicalDomain=network_engine_domain  SubClassName=ps_input  LeftPortType=input  RightPortType=output  PseudoPeriodic=off  Frequencies=[]  NoiseDistribution=none  NoiseParameters=[]  Unit=Pa  AffineConversion=off  FilteringAndDerivatives=zero  SimscapeFilterOrder=1  InputFilterTimeConstant=.001  UdotUserProvided=0
      settings: SourceProductBaseCode=SS,PW,VE
  Conn1 : PMIOPort  Side=Left
  Conn2 : PMIOPort  Port=2  Side=Left
  Conn3 : PMIOPort  Port=3  Side=Right
  Conn4 : PMIOPort  Port=4  Side=Right
  output : Outport
  output1 : Outport  Port=2
  output2 : Outport  Port=3
  output3 : Outport  Port=4
  output4 : Outport  Port=5
  wires:
  PS-Simulink Converter10/1 -> Scope9/1
  input2/1 -> Simulink-PS Converter9/1
  input0/1 -> Simulink-PS Converter7/1
  PS-Simulink Converter9/1 -> output2/1
  input1/1 -> Simulink-PS Converter8/1
  input4/1 -> Simulink-PS Converter6/1
  input3/1 -> Simulink-PS Converter3/1
  PS-Simulink Converter7/1 -> output1/1
  PS-Simulink Converter6/1 -> output4/1
  PS-Simulink Converter5/1 -> output/1
  PS-Simulink Converter8/1 -> output3/1
  connections:
  Simulink-PS Converter8/RConn1 -- DU_SV3_solenoid/LConn1
  HRef Cyl13/LConn1 -- DU_PT2/RConn1
  DU_CV1/LConn2 -- DU_F1/RConn2
  HRef Cyl16/LConn1 -- DU_PT6/RConn1
  PS-Simulink Converter10/LConn1 -- DU_PT6/RConn2
  PS Gain5/RConn1 -- DU_SV3/LConn1
  PS-Simulink Converter6/LConn1 -- DU_PT2/RConn2
  Pipe 6/RConn1 -- DU_SV1/LConn2
  HRef Cyl14/LConn1 -- DU_PT4/RConn1
  Gate Valve/RConn1 -- Pipe 6/LConn1
  Pressure Source2/RConn1 -- PS Gain4/RConn1
  DU_CV2/LConn1 -- PS Gain6/RConn1
  DU_V14/LConn2 -- DU_V1/RConn1
  DU_PT1/LConn1 -- Conn4/RConn1 -- Gate Valve/LConn2
  DU_SV2 Solenoid/RConn1 -- PS Gain6/LConn1
  PS-Simulink Converter9/LConn1 -- DU_PT1/RConn2
  PS Constant13/RConn1 -- DU_V14/LConn1
  DU_V1/LConn1 -- DU_CV2/RConn1
  Simulink-PS Converter9/RConn1 -- DU_SV2 Solenoid/LConn1
  PS Constant12/RConn1 -- DU_V5/LConn1
  PS Constant15/RConn1 -- Gate Valve/LConn1
  PS Gain2/RConn1 -- DU_SV1/LConn1
  Simulink-PS Converter3/RConn1 -- DU_SV1_solenoid/LConn1
  DU_PT2/LConn1 -- Conn2/RConn1 -- DU_V5/RConn1 -- DU_V14/RConn1
  DU_V10/RConn1 -- Gate Valve1/LConn1
  PS-Simulink Converter5/LConn1 -- DU_PT3/RConn2
  DU_SV1_solenoid/RConn1 -- PS Gain2/LConn1
  DU_CV1/RConn1 -- DU_V4/LConn1 -- DU_PT6/LConn1
  HRef Cyl15/LConn1 -- DU_PT1/RConn1
  DU_SV3/RConn1 -- Conn1/RConn1 -- DU_PT4/LConn1
  DU_V5/LConn2 -- DU_V4/RConn1
  Gate Valve1/RConn1 -- DU_CV2/LConn2 -- DU_SV3/LConn2 -- DU_PT3/LConn1
  HRef Cyl11/LConn1 -- DU_PT3/RConn1
  DU_SV1/RConn1 -- DU_F1/LConn1
  Pressure Source2/RConn2 -- HRef Cyl10/LConn1
  DU_SV3_solenoid/RConn1 -- PS Gain5/LConn1
  Simulink-PS Converter6/RConn1 -- DU_SV1_solenoid1/LConn1
  Simulink-PS Converter7/RConn1 -- PS Gain4/LConn1
  DU_F1/RConn1 -- Conn3/RConn1
  PS-Simulink Converter7/LConn1 -- DU_PT4/RConn2
  Gate Valve1/LConn2 -- Pressure Source2/LConn1
  DU_F1/RConn3 -- PS-Simulink Converter8/LConn1
  PS Gain3/RConn1 -- DU_CV1/LConn1
  DU_SV1_solenoid1/RConn1 -- PS Gain3/LConn1

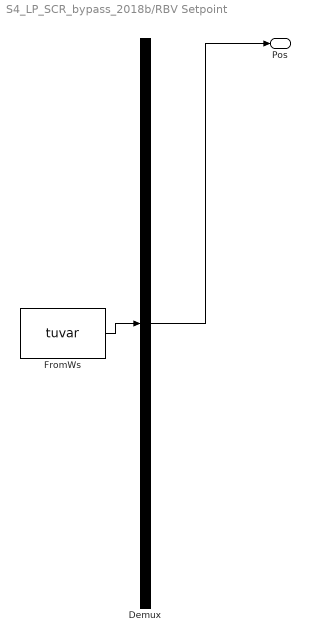
== system S4_LP_SCR_bypass_2018b/RBV Setpoint ==
  Demux : Demux  Tag=STV Demux  Outputs=1
      settings: DisplayOption=none
  FromWs : FromWorkspace  Tag=STV FromWs  VariableName=tuvar
      SigBuilderData=|
      | common.afterFinalStr = 'Extrapolate'
      | common.sampleTime = 0
      | dataSet.timeRange = [0 20000]
      | dataSet.name = 'Group 1'
      | sbobj.Groups.Name = 'Group 1'
      | sbobj.Groups.Signals.Name = 'Pos'
      | sbobj.Groups.Signals.XData = [0 6624 6624 12457 12457 13882 13882 20000]
      | sbobj.Groups.Signals.YData = [1 1 0 0 1 1 0 0]
      | sbobj.Groups.TimeRange = [0 20000]
  Pos : Outport  Tag=STV Outport  VectorParamsAs1DForOutWhenUnconnected=off
  wires:
  Demux/1 -> Pos/1
  FromWs/1 -> Demux/1

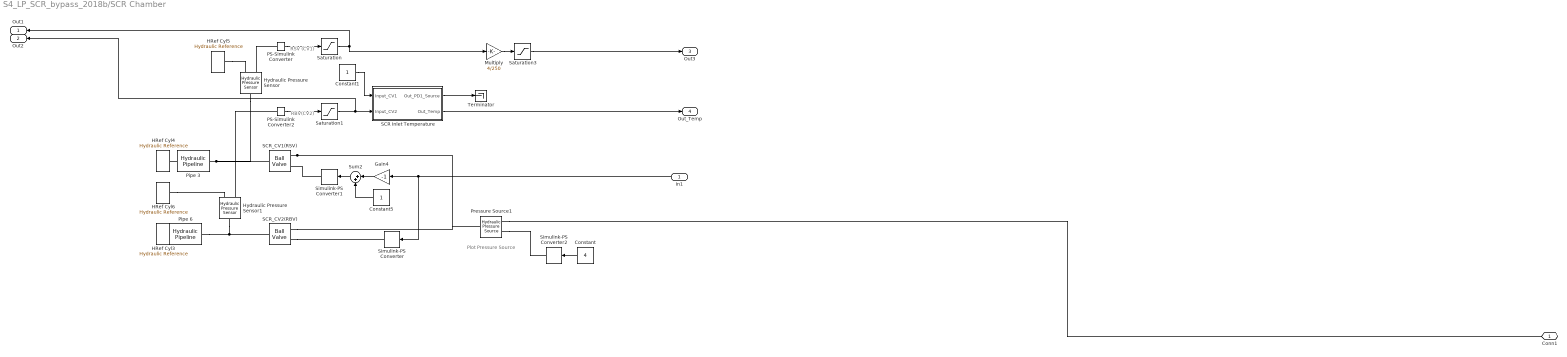
== system S4_LP_SCR_bypass_2018b/SCR Chamber ==
  note: RBV(CV2)
  note: RSV (CV1)
  note: Plot Pressure Source
  In1 : Inport
  Constant : Constant  Value=4
  Constant1 : Constant
  Constant5 : Constant
  Gain4 : Gain  Gain=-1
  HRef Cyl{3..6} (4 alike) : fl_lib/Hydraulic/Hydraulic Elements/Hydraulic Reference  Tag=Factory Generic
      settings: SourceProductBaseCode=PW,SS,VE
  Hydraulic Pressure Sensor : fl_lib/Hydraulic/Hydraulic Sensors/Hydraulic Pressure Sensor
      settings: SourceProductBaseCode=PW,SS,VE
  Hydraulic Pressure Sensor1 : fl_lib/Hydraulic/Hydraulic Sensors/Hydraulic Pressure Sensor
      settings: SourceProductBaseCode=PW,SS,VE
  Multiply : Gain  Gain=4/250
  PS-Simulink Converter : nesl_utility/PS-Simulink Converter  PhysicalDomain=network_engine_domain  SubClassName=ps_output  LeftPortType=input  RightPortType=output  PseudoPeriodic=off  Frequencies=[]  VectorFormat=inherit  Unit=inherit  AffineConversion=off
      settings: SourceProductBaseCode=SS,PW,VE
  PS-Simulink Converter2 : nesl_utility/PS-Simulink Converter  PhysicalDomain=network_engine_domain  SubClassName=ps_output  LeftPortType=input  RightPortType=output  PseudoPeriodic=off  Frequencies=[]  VectorFormat=inherit  Unit=inherit  AffineConversion=off
      settings: SourceProductBaseCode=SS,PW,VE
  Pipe 3 : sh_lib/Pipelines/Hydraulic Pipeline  Tag=Factory Generic  cs_type=1  d_in=0.016 m  area=1e-04 m^2  D_h=0.0112 m  s_factor=500  length=5 m  length_ad=1 m  roughness=1.5e-05 m  Re_lam=2e+03  Re_turb=4e+03  wall_type=1  pr_r_coef=2e-10 m/Pa  time_const=0.008 s  k_sh=1.4  initial_pressure=0 Pa
      settings: SourceProductBaseCode=SH  LogSimulationData=on  InternalSimscapePortConfiguration="{\"Bottom\":[],\"Left\":[{\"id\":\"A\",\"label\":\"A\",\"type\":\"foundation.hydraulic.hydraulic\"}],\"Right\":[{\"id\":\"B\",\"label\":\"B\",\"type\":\"foundation.hydraulic.hydraulic\"}],\"Top\":[]}"
  Pipe 6 : sh_lib/Pipelines/Hydraulic Pipeline  Tag=Factory Generic  cs_type=1  d_in=0.016 m  area=1e-04 m^2  D_h=0.0112 m  s_factor=500  length=5 m  length_ad=1 m  roughness=1.5e-05 m  Re_lam=2e+03  Re_turb=4e+03  wall_type=1  pr_r_coef=2e-10 m/Pa  time_const=0.008 s  k_sh=1.4  initial_pressure=0 Pa
      settings: SourceProductBaseCode=SH  LogSimulationData=on  InternalSimscapePortConfiguration="{\"Bottom\":[],\"Left\":[{\"id\":\"A\",\"label\":\"A\",\"type\":\"foundation.hydraulic.hydraulic\"}],\"Right\":[{\"id\":\"B\",\"label\":\"B\",\"type\":\"foundation.hydraulic.hydraulic\"}],\"Top\":[]}"
  Pressure Source1 : fl_lib/Hydraulic/Hydraulic Sources/Hydraulic Pressure Source  Tag=Factory Generic
      settings: SourceProductBaseCode=PW,SS,VE  InternalSimscapePortConfiguration="{\"Bottom\":[],\"Left\":[{\"id\":\"P\",\"label\":\"P\",\"type\":\"foundation.hydraulic.hydraulic\"}],\"Right\":[{\"id\":\"S\",\"label\":\"S\",\"type\":\"input\"},{\"id\":\"T\",\"label\":\"T\",\"type\":\"foundation.hydraulic.hydraulic\"}],\"Top\":[]}"
  SCR Inlet Temperature : Subsystem
  SCR_CV1(RSV) : sh_lib/Valves/Flow Control Valves/Ball Valve  valve_seat_spec=1  cone_ang=120 deg  d_ball=0.01 m  d_orif=5e-3 m  x_0=0 m  C_d=0.65  A_leak=1e-20 m^2  lam_spec=1  B_lam=0.999  Re_cr=10  flow_rate_specify=off  flow_rate_priority=None  flow_rate=1e-3 m^3/s  flow_rate_nominal_specify=off  flow_rate_nominal_unit=m^3/s  flow_rate_nominal_value=1  pressure_drop_specify=off  pressure_drop_priority=None  pressure_drop=0 Pa  pressure_drop_nominal_specify=off  pressure_drop_nominal_unit=Pa  pressure_drop_nominal_value=1
      settings: SourceProductBaseCode=SH  InternalSimscapePortConfiguration="{\"Bottom\":[],\"Left\":[{\"id\":\"S\",\"label\":\"S\",\"type\":\"input\"},{\"id\":\"A\",\"label\":\"A\",\"type\":\"foundation.hydraulic.hydraulic\"}],\"Right\":[{\"id\":\"B\",\"label\":\"B\",\"type\":\"foundation.hydraulic.hydraulic\"}],\"Top\":[]}"
  SCR_CV2(RBV) : sh_lib/Valves/Flow Control Valves/Ball Valve  valve_seat_spec=1  cone_ang=120 deg  d_ball=0.01 m  d_orif=5e-3 m  x_0=0 m  C_d=0.65  A_leak=1e-20 m^2  lam_spec=1  B_lam=0.999  Re_cr=10  flow_rate_specify=off  flow_rate_priority=None  flow_rate=1e-3 m^3/s  flow_rate_nominal_specify=off  flow_rate_nominal_unit=m^3/s  flow_rate_nominal_value=1  pressure_drop_specify=off  pressure_drop_priority=None  pressure_drop=0 Pa  pressure_drop_nominal_specify=off  pressure_drop_nominal_unit=Pa  pressure_drop_nominal_value=1
      settings: SourceProductBaseCode=SH  InternalSimscapePortConfiguration="{\"Bottom\":[],\"Left\":[{\"id\":\"S\",\"label\":\"S\",\"type\":\"input\"},{\"id\":\"A\",\"label\":\"A\",\"type\":\"foundation.hydraulic.hydraulic\"}],\"Right\":[{\"id\":\"B\",\"label\":\"B\",\"type\":\"foundation.hydraulic.hydraulic\"}],\"Top\":[]}"
  Saturation : Saturate  UpperLimit=1  LowerLimit=0
  Saturation1 : Saturate  UpperLimit=1  LowerLimit=0
  Saturation3 : Saturate  UpperLimit=inf  LowerLimit=0
  Simulink-PS Converter : nesl_utility/Simulink-PS Converter  PhysicalDomain=network_engine_domain  SubClassName=ps_input  LeftPortType=input  RightPortType=output  PseudoPeriodic=off  Frequencies=[]  NoiseDistribution=none  NoiseParameters=[]  Unit=m  AffineConversion=off  FilteringAndDerivatives=zero  SimscapeFilterOrder=1  InputFilterTimeConstant=.001  UdotUserProvided=0
      settings: SourceProductBaseCode=SS,PW,VE
  Simulink-PS Converter1 : nesl_utility/Simulink-PS Converter  PhysicalDomain=network_engine_domain  SubClassName=ps_input  LeftPortType=input  RightPortType=output  PseudoPeriodic=off  Frequencies=[]  NoiseDistribution=none  NoiseParameters=[]  Unit=m  AffineConversion=off  FilteringAndDerivatives=zero  SimscapeFilterOrder=1  InputFilterTimeConstant=.001  UdotUserProvided=0
      settings: SourceProductBaseCode=SS,PW,VE
  Simulink-PS Converter2 : nesl_utility/Simulink-PS Converter  PhysicalDomain=network_engine_domain  SubClassName=ps_input  LeftPortType=input  RightPortType=output  PseudoPeriodic=off  Frequencies=[]  NoiseDistribution=none  NoiseParameters=[]  Unit=Pa  AffineConversion=off  FilteringAndDerivatives=zero  SimscapeFilterOrder=1  InputFilterTimeConstant=.001  UdotUserProvided=0
      settings: SourceProductBaseCode=SS,PW,VE
  Sum2 : Sum  Inputs=|++
  Terminator : Terminator
  Conn1 : PMIOPort  Side=Right
  Out1 : Outport
  Out2 : Outport  Port=2
  Out3 : Outport  Port=3
  Out_Temp : Outport  Port=4
  wires:
  Constant/1 -> Simulink-PS Converter2/1
  Saturation/1 -> Multiply/1, Out1/1
  Saturation1/1 -> Out2/1, SCR Inlet Temperature/2(Input_CV2)
  PS-Simulink Converter2/1 -> Saturation1/1
  Gain4/1 -> Sum2/1
  Multiply/1 -> Saturation3/1
  Constant5/1 -> Sum2/2
  Saturation3/1 -> Out3/1
  Sum2/1 -> Simulink-PS Converter1/1
  PS-Simulink Converter/1 -> Saturation/1
  In1/1 -> Simulink-PS Converter/1, Gain4/1
  SCR Inlet Temperature/2(Out_Temp) -> Out_Temp/1
  SCR Inlet Temperature/1(Out_PD1_Source) -> Terminator/1
  Constant1/1 -> SCR Inlet Temperature/1(Input_CV1)
  connections:
  HRef Cyl5/LConn1 -- Hydraulic Pressure Sensor/RConn1
  Simulink-PS Converter1/RConn1 -- SCR_CV1(RSV)/LConn1
  HRef Cyl6/LConn1 -- Hydraulic Pressure Sensor1/RConn1
  PS-Simulink Converter/LConn1 -- Hydraulic Pressure Sensor/RConn2
  Pipe 6/RConn1 -- HRef Cyl3/LConn1
  Pipe 3/RConn1 -- HRef Cyl4/LConn1
  Pressure Source1/RConn2 -- Conn1/RConn1
  Pipe 3/LConn1 -- Hydraulic Pressure Sensor/LConn1 -- SCR_CV1(RSV)/RConn1
  SCR_CV1(RSV)/LConn2 -- SCR_CV2(RBV)/LConn2 -- Pressure Source1/LConn1
  Hydraulic Pressure Sensor1/LConn1 -- SCR_CV2(RBV)/RConn1 -- Pipe 6/LConn1
  Pressure Source1/RConn1 -- Simulink-PS Converter2/RConn1
  SCR_CV2(RBV)/LConn1 -- Simulink-PS Converter/RConn1
  PS-Simulink Converter2/LConn1 -- Hydraulic Pressure Sensor1/RConn2

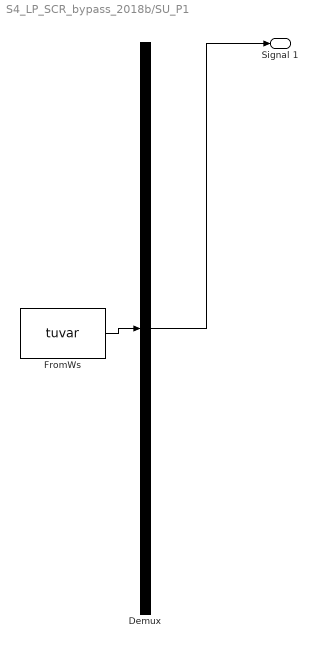
== system S4_LP_SCR_bypass_2018b/SU_P1 ==
  Demux : Demux  Tag=STV Demux  Outputs=1
      settings: DisplayOption=none
  FromWs : FromWorkspace  Tag=STV FromWs  VariableName=tuvar
      SigBuilderData=|
      | common.afterFinalStr = 'Extrapolate'
      | common.sampleTime = 0
      | dataSet.timeRange = [0 20000]
      | dataSet.name = 'Group 1'
      | sbobj.Groups.Name = 'Group 1'
      | sbobj.Groups.Signals.Name = 'Signal 1'
      | sbobj.Groups.Signals.XData = [0 1408 1408 1900 1900 5370 5370 12429 12429 16094 16094 18499 18499 20000]
      | sbobj.Groups.Signals.YData = [0 0 1 1 0 0 1 1 0 0 1 1 0 0]
      | sbobj.Groups.TimeRange = [0 20000]
  Signal 1 : Outport  Tag=STV Outport
  wires:
  Demux/1 -> Signal 1/1
  FromWs/1 -> Demux/1

== system S4_LP_SCR_bypass_2018b/SU_P2 ==
  Demux : Demux  Tag=STV Demux  Outputs=1
      settings: DisplayOption=none
  FromWs : FromWorkspace  Tag=STV FromWs  VariableName=tuvar
      SigBuilderData=|
      | common.afterFinalStr = 'Extrapolate'
      | common.sampleTime = 0
      | dataSet.timeRange = [0 20000]
      | dataSet.name = 'Group 1'
      | sbobj.Groups.Name = 'Group 1'
      | sbobj.Groups.Signals.Name = 'Signal 1'
      | sbobj.Groups.Signals.XData = [0 20000]
      | sbobj.Groups.Signals.YData = [0 0]
      | sbobj.Groups.TimeRange = [0 20000]
  Signal 1 : Outport  Tag=STV Outport
  wires:
  Demux/1 -> Signal 1/1
  FromWs/1 -> Demux/1
